simulink model "model"  (R2022b)
settings: Solver=VariableStepAuto  StartTime=0.0  StopTime=30  RelTol=1e-3
settings Model: Creator=26083  LastModifiedBy=AWWOLF

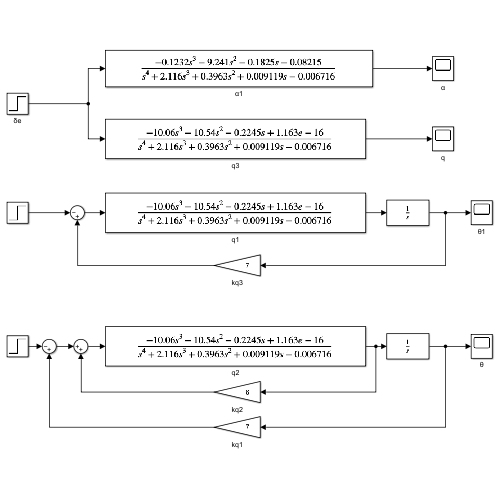
[thumbnail: Simulink's stored preview of the top-level diagram]
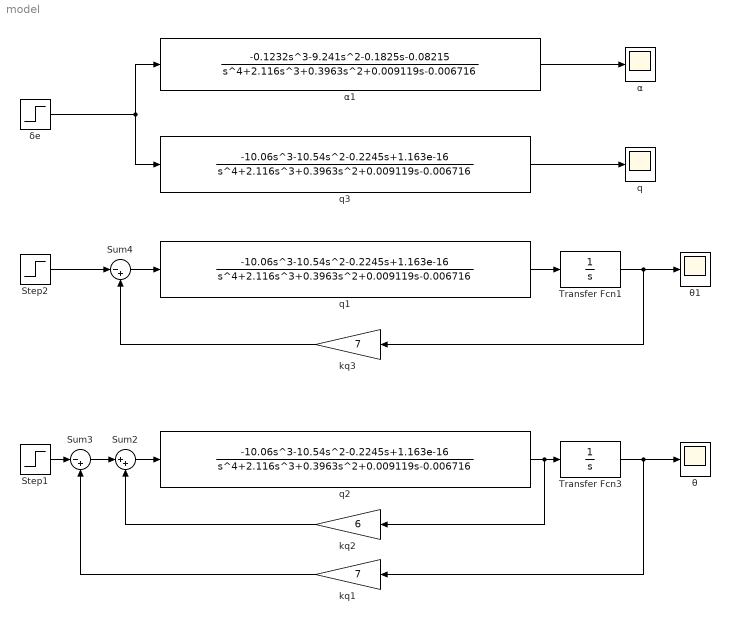
== system model ==
  Step1 : Step  SampleTime=0
  Step2 : Step  SampleTime=0
  Sum2 : Sum  Inputs=|++
  Sum3 : Sum  Inputs=|-+
  Sum4 : Sum  Inputs=|-+
  Transfer Fcn1 : TransferFcn  Denominator=[1 0]
  Transfer Fcn3 : TransferFcn  Denominator=[1 0]
  kq1 : Gain  Gain=7
  kq2 : Gain  Gain=6
  kq3 : Gain  Gain=7
  q : Scope
  q1 : TransferFcn  Numerator=[-10.06 -10.54 -0.2245 1.163e-16]  Denominator=[1 2.116 0.3963 0.009119 -0.006716]
  q2 : TransferFcn  Numerator=[-10.06 -10.54 -0.2245 1.163e-16]  Denominator=[1 2.116 0.3963 0.009119 -0.006716]
  q3 : TransferFcn  Numerator=[-10.06 -10.54 -0.2245 1.163e-16]  Denominator=[1 2.116 0.3963 0.009119 -0.006716]
  α : Scope
  α1 : TransferFcn  Numerator=[-0.1232 -9.241 -0.1825 -0.08215]  Denominator=[1 2.116 0.3963 0.009119 -0.006716]
  δe : Step  SampleTime=0
  θ : Scope
  θ1 : Scope
  wires:
  Transfer Fcn3/1 -> kq1/1, θ/1
  Step1/1 -> Sum3/1
  q2/1 -> kq2/1, Transfer Fcn3/1
  kq1/1 -> Sum3/2
  Sum3/1 -> Sum2/1
  Sum2/1 -> q2/1
  kq2/1 -> Sum2/2
  δe/1 -> q3/1, α1/1
  α1/1 -> α/1
  q3/1 -> q/1
  Transfer Fcn1/1 -> kq3/1, θ1/1
  Step2/1 -> Sum4/1
  kq3/1 -> Sum4/2
  q1/1 -> Transfer Fcn1/1
  Sum4/1 -> q1/1
